simulink model "senza_cascata_discreto"  (R2019b)
settings: Solver=VariableStepAuto  StartTime=0.0  StopTime=10  RelTol=1e-3
undefined symbols (not defined in the file or in its folder): den_G1, den_G2, den_Raa, DENd, DENpf, num_G1, num_G2, num_Raa, NUMd, NUMpf, Ts
settings Model: Creator=edoardo  LastModifiedBy=edoardo

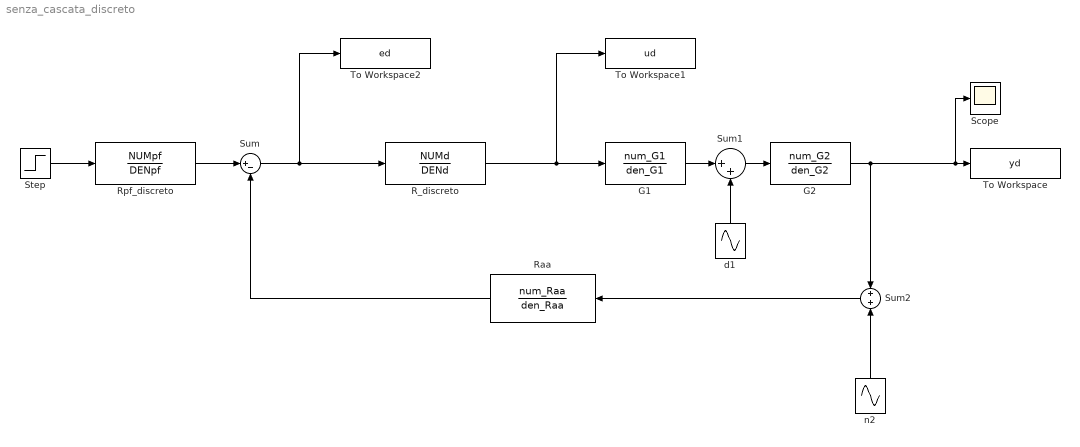
== system senza_cascata_discreto ==
  "G1 " : TransferFcn  Numerator=num_G1  Denominator=den_G1
  G2 : TransferFcn  Numerator=num_G2  Denominator=den_G2
  "R_discreto " : DiscreteTransferFcn  Numerator=NUMd  Denominator=DENd  SampleTime=Ts
  Raa : TransferFcn  Numerator=num_Raa  Denominator=den_Raa
  "Rpf_discreto " : DiscreteTransferFcn  Numerator=NUMpf  Denominator=DENpf  SampleTime=Ts
  Scope : Scope
  Step : Step  Time=0  After=1.5  SampleTime=0
  Sum : Sum  Inputs=|+-
  Sum1 : Sum  Inputs=|++
  Sum2 : Sum
  To Workspace : ToWorkspace  VariableName=yd  SaveFormat=Timeseries  SampleTime=-1
  To Workspace1 : ToWorkspace  VariableName=ud  SaveFormat=Timeseries  SampleTime=-1
  To Workspace2 : ToWorkspace  VariableName=ed  SaveFormat=Timeseries  SampleTime=-1
  d1 : Sin  Amplitude=3  SampleTime=0
  n2 : Sin  Amplitude=0.02  Frequency=8000  SampleTime=0
  wires:
  Step/1 -> "Rpf_discreto "/1
  Sum1/1 -> G2/1
  d1/1 -> Sum1/2
  "G1 "/1 -> Sum1/1
  Sum/1 -> "R_discreto "/1, To Workspace2/1
  "R_discreto "/1 -> To Workspace1/1, "G1 "/1
  G2/1 -> Sum2/1, Scope/1, To Workspace/1
  "Rpf_discreto "/1 -> Sum/1
  n2/1 -> Sum2/2
  Sum2/1 -> Raa/1
  Raa/1 -> Sum/2
